simulink model "Planar2L"  (R2018a)
settings: Solver=VariableStepAuto  StartTime=0.0  StopTime=td  RelTol=1e-3
values from neighbouring files (symbols this model uses):
  KDgrav = diag([kd1 kd2])    [Parameters.m]    (also in modifyg.m)
  KPgrav = diag([kp1 kp2])    [Parameters.m]    (also in modifyg.m)
  qdgrav = input('')    [Parameters.m]
  qigrav = input('')    [Parameters.m]
  tc = input('')    [Parameters.m]    (also in modifyg.m = V)
undefined symbols (not defined in the file or in its folder): c11, c12, c21, Fv, G1a, G1b, G2, InertiaMatrix
settings Model: Creator=Amr  LastModifiedBy=Amr

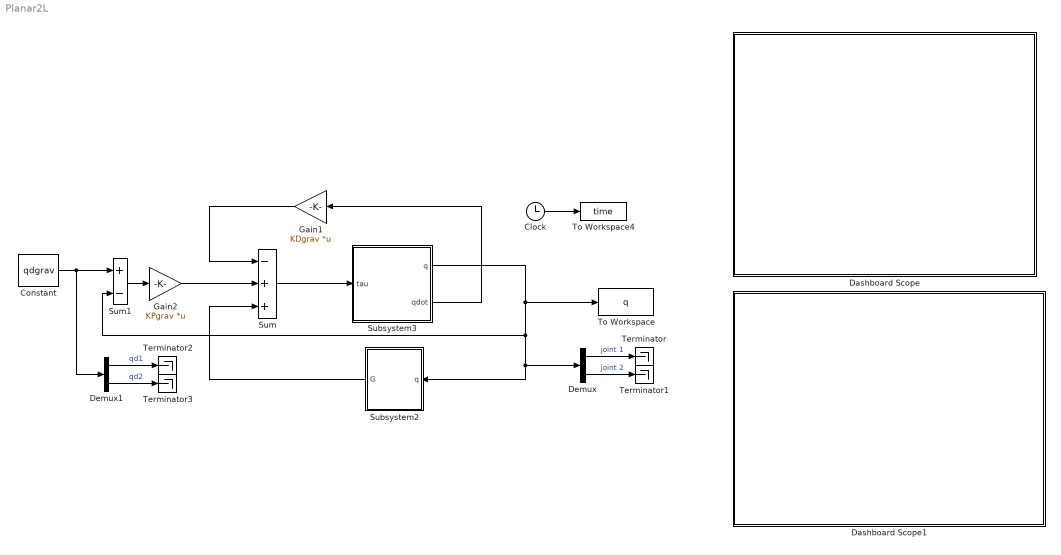
== system Planar2L ==
  Clock : Clock
  Constant : Constant  Value=qdgrav
  Dashboard Scope : Subsystem  DialogController=hmiCreateDDGDialog  IsWebBlock=on  mask(MWDashboardBlock){webBlockId=75545e27-693e-49e5-a9e5-8890266f6020, webBlockType=sdiscope, ShowInitialText=on, HMISrcModelName=Planar2L}
      mask prompts: webBlockId "WebBlock Id"; webBlockType "WebBlock Type"; HMISrcModelName "Source Model"
      mask help: SimulinkHMI:dialogs:HMIScopeDialogDesc
      mask Help: helpview([docroot '/mapfiles/simulink.map'], 'hmi_scope')
      mask Display:
      | if strcmp(get_param(bdroot(gcb),'BlockDiagramType'), 'library')
      |     image([(matlabroot) '/toolbox/simulink/hmi/icons/DashboardScope.png']);
      | end
  Dashboard Scope1 : Subsystem  DialogController=hmiCreateDDGDialog  IsWebBlock=on  mask(MWDashboardBlock){webBlockId=ee8584ce-b275-49de-b7cd-f82f21c12e6e, webBlockType=sdiscope, ShowInitialText=on, HMISrcModelName=Planar2L}
      mask prompts: webBlockId "WebBlock Id"; webBlockType "WebBlock Type"; HMISrcModelName "Source Model"
      mask help: SimulinkHMI:dialogs:HMIScopeDialogDesc
      mask Help: helpview([docroot '/mapfiles/simulink.map'], 'hmi_scope')
      mask Display:
      | if strcmp(get_param(bdroot(gcb),'BlockDiagramType'), 'library')
      |     image([(matlabroot) '/toolbox/simulink/hmi/icons/DashboardScope.png']);
      | end
  Demux : Demux  Outputs=2
  Demux1 : Demux  Outputs=2
  Gain1 : Gain  Gain=KDgrav  Multiplication=Matrix(K*u)  SampleTime=tc
      mask Display: disp('KD')
  Gain2 : Gain  Gain=KPgrav  Multiplication=Matrix(K*u)  SampleTime=tc
      mask Display: disp('KP')
  Subsystem2 : Subsystem
      mask Display: disp('g(q)')
  Subsystem3 : Subsystem
      mask Display: disp('Manipulator')
  Sum : Sum  Inputs=-++
  Sum1 : Sum  Inputs=+-
  Terminator{,1..3} (4 alike) : Terminator
  To Workspace : ToWorkspace  VariableName=q  SampleTime=tc
      settings: MaxDataPoints=4001
  To Workspace4 : ToWorkspace  VariableName=time  SampleTime=tc
      settings: MaxDataPoints=4001
  wires:
  Gain2/1 -> Sum/2
  Subsystem2/1(G) -> Sum/3
  Sum/1 -> Subsystem3/1(tau)
  Gain1/1 -> Sum/1
  Sum1/1 -> Gain2/1
  Subsystem3/2(qdot) -> Gain1/1
  Subsystem3/1(q) -> To Workspace/1, Demux/1, Subsystem2/1(q), Sum1/2
  Constant/1 -> Demux1/1, Sum1/1
  Clock/1 -> To Workspace4/1
  Demux/1 -> Terminator/1  "joint 1"
  Demux/2 -> Terminator1/1  "joint 2"
  Demux1/1 -> Terminator2/1  "qd1"
  Demux1/2 -> Terminator3/1  "qd2"

== system Planar2L/Dashboard Scope ==

== system Planar2L/Dashboard Scope1 ==

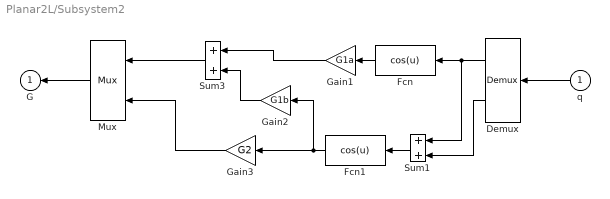
== system Planar2L/Subsystem2 ==
  q : Inport
  Demux : Demux  Outputs=2
      mask Display: disp('Demux')
  Fcn : Fcn  Expr=cos(u)
  Fcn1 : Fcn  Expr=cos(u)
  Gain1 : Gain  Gain=G1a
      mask Display: disp('G1a')
  Gain2 : Gain  Gain=G1b
      mask Display: disp('G1b')
  Gain3 : Gain  Gain=G2
      mask Display: disp('G2')
  Mux : Mux  Inputs=2
      mask Display: disp('Mux')
  Sum1 : Sum  SampleTime=tc  SaturateOnIntegerOverflow=on  InputSameDT=on  OutDataTypeStr=Inherit: Same as first input
  Sum3 : Sum  SampleTime=tc  SaturateOnIntegerOverflow=on  InputSameDT=on  OutDataTypeStr=Inherit: Same as first input
  G : Outport
  wires:
  Fcn/1 -> Gain1/1
  Demux/1 -> Sum1/1, Fcn/1
  Fcn1/1 -> Gain3/1, Gain2/1
  Gain3/1 -> Mux/2
  Sum1/1 -> Fcn1/1
  Sum3/1 -> Mux/1
  Mux/1 -> G/1
  q/1 -> Demux/1
  Demux/2 -> Sum1/2
  Gain1/1 -> Sum3/1
  Gain2/1 -> Sum3/2

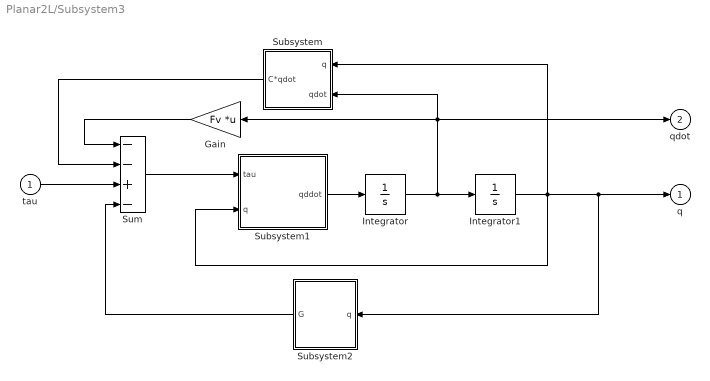
== system Planar2L/Subsystem3 ==
  tau : Inport
  Gain : Gain  Gain=Fv  Multiplication=Matrix(K*u)
      mask Display: disp('Friction')
  Integrator : Integrator  InitialCondition=[0 0]
  Integrator1 : Integrator  InitialCondition=qigrav
  Subsystem : Subsystem
      mask Display: disp('C*qdot')
  Subsystem1 : Subsystem
      mask Display: disp('inv(B(q))*tau')
  Subsystem2 : Subsystem
      mask Display: disp('g(q)')
  Sum : Sum  Inputs=--+-
  q : Outport
  qdot : Outport  Port=2
  wires:
  Gain/1 -> Sum/1
  Integrator/1 -> qdot/1, Gain/1, Subsystem/2(qdot), Integrator1/1
  Subsystem1/1(qddot) -> Integrator/1
  Integrator1/1 -> q/1, Subsystem2/1(q), Subsystem1/2(q), Subsystem/1(q)
  tau/1 -> Sum/3
  Subsystem2/1(G) -> Sum/4
  Subsystem/1(C*qdot) -> Sum/2
  Sum/1 -> Subsystem1/1(tau)

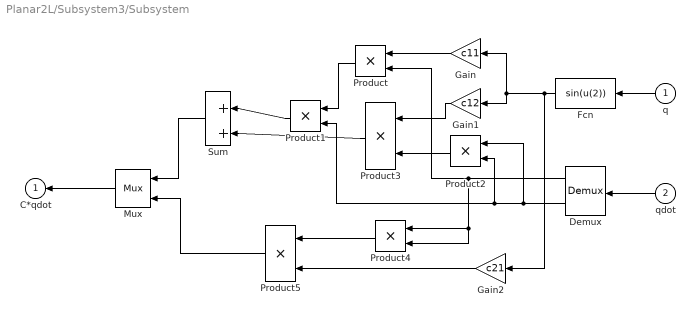
== system Planar2L/Subsystem3/Subsystem ==
  q : Inport
  qdot : Inport  Port=2
  Demux : Demux  Outputs=2
      mask Display: disp('Demux')
  Fcn : Fcn  Expr=sin(u(2))
  Gain : Gain  Gain=c11
      mask Display: disp('c11')
  Gain1 : Gain  Gain=c12
      mask Display: disp('c12')
  Gain2 : Gain  Gain=c21
      mask Display: disp('c21')
  Mux : Mux  Inputs=2
      mask Display: disp('Mux')
  Product{,1..5} (6 alike) : Product
  Sum : Sum  Inputs=|++
  C*qdot : Outport
  wires:
  Demux/2 -> Product2/2, Product1/2, Product2/1
  Sum/1 -> Mux/1
  Product5/1 -> Mux/2
  Demux/1 -> Product/2, Product4/1, Product4/2
  Product4/1 -> Product5/1
  Fcn/1 -> Gain2/1, Gain1/1, Gain/1
  Gain2/1 -> Product5/2
  Product2/1 -> Product3/2
  Product1/1 -> Sum/1
  Product/1 -> Product1/1
  q/1 -> Fcn/1
  Gain1/1 -> Product3/1
  Product3/1 -> Sum/2
  qdot/1 -> Demux/1
  Mux/1 -> C*qdot/1
  Gain/1 -> Product/1

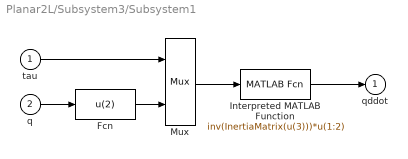
== system Planar2L/Subsystem3/Subsystem1 ==
  tau : Inport
  q : Inport  Port=2
  Fcn : Fcn  Expr=u(2)
  Interpreted MATLAB Function : MATLABFcn  MATLABFcn=inv(InertiaMatrix(u(3)))*u(1:2)  OutputDimensions=2
  Mux : Mux  Inputs=[2,1]
      mask Display: disp('Mux')
  qddot : Outport
  wires:
  Mux/1 -> Interpreted MATLAB Function/1
  Interpreted MATLAB Function/1 -> qddot/1
  q/1 -> Fcn/1
  tau/1 -> Mux/1
  Fcn/1 -> Mux/2

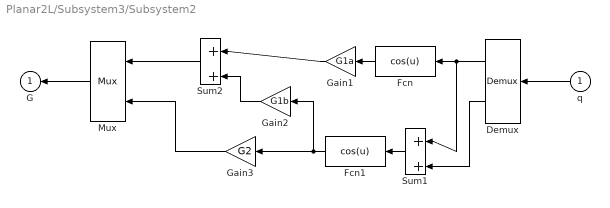
== system Planar2L/Subsystem3/Subsystem2 ==
  q : Inport
  Demux : Demux  Outputs=2
      mask Display: disp('Demux')
  Fcn : Fcn  Expr=cos(u)
  Fcn1 : Fcn  Expr=cos(u)
  Gain1 : Gain  Gain=G1a
      mask Display: disp('G1a')
  Gain2 : Gain  Gain=G1b
      mask Display: disp('G1b')
  Gain3 : Gain  Gain=G2
      mask Display: disp('G2')
  Mux : Mux  Inputs=2
      mask Display: disp('Mux')
  Sum1 : Sum  Inputs=|++
  Sum2 : Sum  Inputs=|++
  G : Outport
  wires:
  Gain2/1 -> Sum2/2
  Fcn/1 -> Gain1/1
  Gain1/1 -> Sum2/1
  Demux/1 -> Fcn/1, Sum1/1
  Fcn1/1 -> Gain3/1, Gain2/1
  Gain3/1 -> Mux/2
  Demux/2 -> Sum1/2
  Sum1/1 -> Fcn1/1
  Sum2/1 -> Mux/1
  Mux/1 -> G/1
  q/1 -> Demux/1
